simulink library "sensorProcessing_lib"  (R2018b)
settings: Solver=VariableStepAuto  StartTime=0.0  StopTime=10.0  RelTol=1e-3
undefined symbols (not defined in the file or in its folder): fswParams
libraries: maggyroProcessing_lib x2, mag_mtq_duty_cycle_lib x1, pd_processing_lib x1, sunsensor_processing_lib x1
settings Model: Creator=kylle  LastModifiedBy=aact_

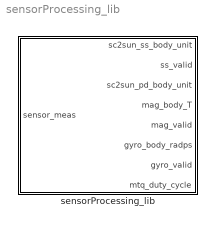
== system sensorProcessing_lib ==
  sensorProcessing_lib : Subsystem  TreatAsAtomicUnit=on

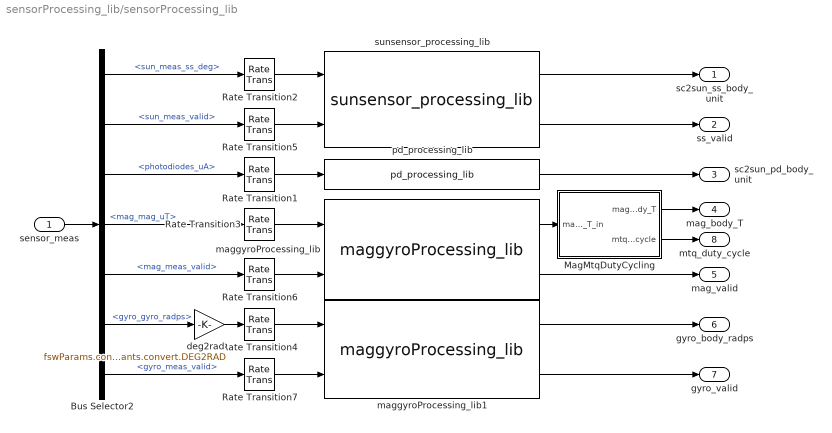
== system sensorProcessing_lib/sensorProcessing_lib ==
  sensor_meas : Inport  OutDataTypeStr=Bus: sensor_bus
  Bus Selector2 : BusSelector  OutputSignals=sun_meas_ss_deg,sun_meas_valid,photodiodes_uA,mag_mag_uT,mag_meas_valid,gyro_gyro_radps,gyro_meas_valid
  MagMtqDutyCycling : Subsystem
  Rate Transition{1..7} (7 alike) : RateTransition  OutPortSampleTime=fswParams.sample_time_s
  deg2rad : Gain  Gain=fswParams.constants.convert.DEG2RAD
  maggyroProcessing_lib : maggyroProcessing_lib/maggyroProcessing_lib  static_range_max_value=fswParams.sensors.mag_static_range  offset_calibration_matrix=fswParams.sensors.mag_offset  max_err=fswParams.sensors.mag_max_err  rotation_calibration_matrix=fswParams.sensors.mag_rotate  Gain=fswParams.constants.convert.uT2T
  maggyroProcessing_lib1 : maggyroProcessing_lib/maggyroProcessing_lib  static_range_max_value=fswParams.sensors.gyro_static_range  offset_calibration_matrix=fswParams.sensors.gyro_offset  max_err=fswParams.sensors.gyro_max_err  rotation_calibration_matrix=fswParams.sensors.gyro_rotate  Gain=1
  pd_processing_lib : pd_processing_lib/pd_processing_lib  SystemSampleTime=-1
  sunsensor_processing_lib : sunsensor_processing_lib/sunsensor_processing_lib  SystemSampleTime=-1
  sc2sun_ss_body_unit : Outport
  ss_valid : Outport  Port=2
  sc2sun_pd_body_unit : Outport  Port=3
  mag_body_T : Outport  Port=4
  mag_valid : Outport  Port=5
  gyro_body_radps : Outport  Port=6
  gyro_valid : Outport  Port=7
  mtq_duty_cycle : Outport  Port=8
  wires:
  Bus Selector2/2 -> Rate Transition5/1  "<sun_meas_valid>"
  sensor_meas/1 -> Bus Selector2/1
  Bus Selector2/7 -> Rate Transition7/1  "<gyro_meas_valid>"
  Bus Selector2/5 -> Rate Transition6/1  "<mag_meas_valid>"
  sunsensor_processing_lib/1 -> sc2sun_ss_body_unit/1
  Bus Selector2/4 -> Rate Transition3/1  "<mag_mag_uT>"
  Bus Selector2/1 -> Rate Transition2/1  "<sun_meas_ss_deg>"
  Bus Selector2/6 -> deg2rad/1  "<gyro_gyro_radps>"
  maggyroProcessing_lib1/2 -> gyro_valid/1
  maggyroProcessing_lib/2 -> mag_valid/1
  maggyroProcessing_lib1/1 -> gyro_body_radps/1
  sunsensor_processing_lib/2 -> ss_valid/1
  Bus Selector2/3 -> Rate Transition1/1  "<photodiodes_uA>"
  pd_processing_lib/1 -> sc2sun_pd_body_unit/1
  Rate Transition2/1 -> sunsensor_processing_lib/1
  Rate Transition1/1 -> pd_processing_lib/1
  Rate Transition3/1 -> maggyroProcessing_lib/1
  Rate Transition4/1 -> maggyroProcessing_lib1/1
  Rate Transition5/1 -> sunsensor_processing_lib/2
  Rate Transition6/1 -> maggyroProcessing_lib/2
  Rate Transition7/1 -> maggyroProcessing_lib1/2
  maggyroProcessing_lib/1 -> MagMtqDutyCycling/1(mag_body_T_in)
  MagMtqDutyCycling/1(mag_body_T) -> mag_body_T/1
  MagMtqDutyCycling/2(mtq_duty_cycle) -> mtq_duty_cycle/1
  deg2rad/1 -> Rate Transition4/1

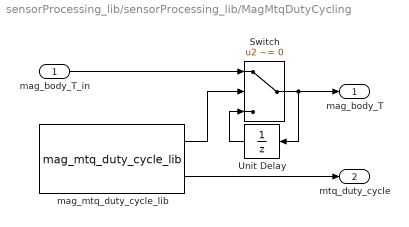
== system sensorProcessing_lib/sensorProcessing_lib/MagMtqDutyCycling ==
  mag_body_T_in : Inport
  Switch : Switch  Criteria=u2 ~= 0  OutDataTypeStr=double  InputSameDT=on
  Unit Delay : UnitDelay  InitialCondition=[0;0;1]  SampleTime=-1
  mag_mtq_duty_cycle_lib : mag_mtq_duty_cycle_lib/mag_mtq_duty_cycle_lib  SystemSampleTime=-1
  mag_body_T : Outport
  mtq_duty_cycle : Outport  Port=2
  wires:
  mag_mtq_duty_cycle_lib/1 -> Switch/2
  mag_mtq_duty_cycle_lib/2 -> mtq_duty_cycle/1
  mag_body_T_in/1 -> Switch/1
  Unit Delay/1 -> Switch/3
  Switch/1 -> Unit Delay/1, mag_body_T/1
